simulink model "sim_final"  (R2023b)
settings: Solver=FixedStepAuto  StartTime=0.0  StopTime=10.0  RelTol=1e-3  EnableMultiTasking=on
libraries: raspberrypiAVlib x1
settings Model: Creator=Admin  LastModifiedBy=Admin
settings SolverCC: PositivePriorityOrder=on
settings OptimizationCC: EnhancedBackFolding=on  PassReuseOutputArgsAs=Individual arguments  ZeroExternalMemoryAtStartup=off  ZeroInternalMemoryAtStartup=off  MaxStackSize=64  OptimizeBlockOrder=speed  DifferentSizesBufferReuse=on  OptimizationCustomize=off  EfficientTunableParamExpr=on
settings DebuggingCC: ParameterTunabilityLossMsg=error
settings HardwareCC: ProdBitPerPointer=32  ProdBitPerSizeT=32  ProdBitPerPtrDiffT=32  ProdLargestAtomicInteger=Long  ProdLargestAtomicFloat=Double  ProdWordSize=32  ProdLongLongMode=on  ProdHWDeviceType=ARM Compatible->ARM Cortex  UseEmbeddedCoderFeatures=off  UseSimulinkCoderFeatures=off
settings RTWCC: Description=Embedded Coder  SystemTargetFile=ert.tlc  HardwareBoard=Raspberry Pi  TLCOptions="-aInlineSetEventsForThisBaseRateFcn=TLC_FALSE -aSuppressMultiTaskScheduler=TLC_FALSE  -aRateBasedStepFcn=0"  TemplateMakefile=ert_default_tmf  Toolchain=GNU GCC Embedded Linux  BuildConfiguration=Faster Runs
settings CodeAppCC: ForceParamTrailComments=on  IgnoreCustomStorageClasses=off  OperatorAnnotations=on  SimulinkDataObjDesc=on  SFDataObjDesc=on  InsertBlockDesc=on
settings ERTTargetCC: SupportNonInlinedSFcns=on  SupportVariableSizeSignals=on  ExtModeTransport=2  ExtModeStaticAlloc=on  ExtModeMexFile=ext_xcp  ExtModeIntrfLevel=Level2 - Open

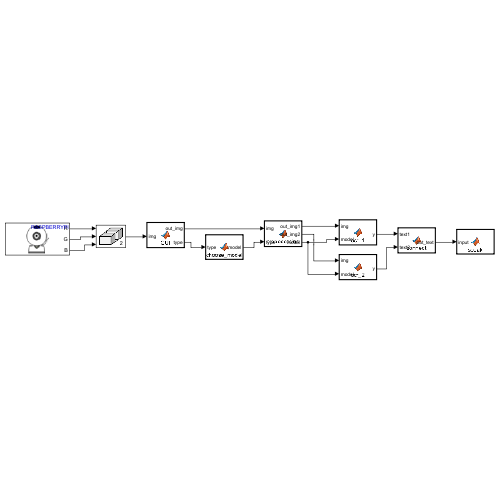
[thumbnail: Simulink's stored preview of the top-level diagram]
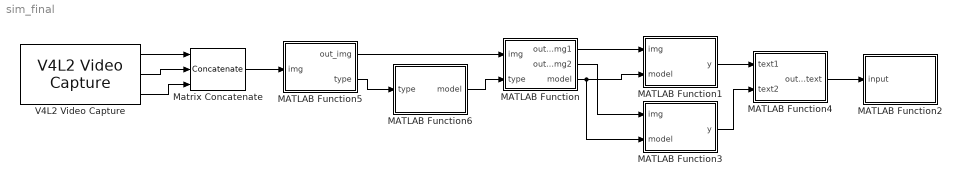
== system sim_final ==
  MATLAB Function : MATLAB Function  TreatAsAtomicUnit=on
  MATLAB Function1 : MATLAB Function  TreatAsAtomicUnit=on
  MATLAB Function2 : MATLAB Function  TreatAsAtomicUnit=on
  MATLAB Function3 : MATLAB Function  TreatAsAtomicUnit=on
  MATLAB Function4 : MATLAB Function  TreatAsAtomicUnit=on
  MATLAB Function5 : MATLAB Function  TreatAsAtomicUnit=on
  MATLAB Function6 : MATLAB Function  TreatAsAtomicUnit=on
  Matrix Concatenate : Concatenate  NumInputs=3  Mode=Multidimensional array  ConcatenateDimension=2
  V4L2 Video Capture : raspberrypiAVlib/V4L2 Video Capture  DeviceName=/dev/video0  Resolution=320x240  CustomResolution=[ 320, 240 ]  PixelFormat=RGB  SampleTime=0.1  pixelOrder=planar  simOutput=Colorbars  imSizeSelection=320x240  imSize=[640, 480]  roi=[0, 0, 640, 480]  m_devName='/dev/video0'  blockPlatform=LINUX  HorizontalFlip=off  VerticalFlip=off  Brightness=0.5  Saturation=0.5  Contrast=0.5  Sharpness=0.5  CameraPan=0  CameraTilt=0  CameraZoom=0.5  EnableManualFocus=on  ManualFocus=0.5
  wires:
  MATLAB Function/1(out_img1) -> MATLAB Function1/1(img)
  MATLAB Function5/2(type) -> MATLAB Function6/1(type)
  V4L2 Video Capture/1 -> Matrix Concatenate/1
  V4L2 Video Capture/2 -> Matrix Concatenate/2
  V4L2 Video Capture/3 -> Matrix Concatenate/3
  Matrix Concatenate/1 -> MATLAB Function5/1(img)
  MATLAB Function/2(out_img2) -> MATLAB Function3/1(img)
  MATLAB Function6/1(model) -> MATLAB Function/2(type)
  MATLAB Function5/1(out_img) -> MATLAB Function/1(img)
  MATLAB Function/3(model) -> MATLAB Function1/2(model), MATLAB Function3/2(model)
  MATLAB Function1/1(y) -> MATLAB Function4/1(text1)
  MATLAB Function3/1(y) -> MATLAB Function4/2(text2)
  MATLAB Function4/1(out_text) -> MATLAB Function2/1(input)

== matlab function sim_final/MATLAB Function1 ==
  data: img input; y output; model input
function y = ocr_1(img,model)

y = img;

== matlab function sim_final/MATLAB Function ==
  data: img input; out_img1 output; out_img2 output; type input; model output
function [out_img1,out_img2,model] = prepocessing(img,type)

out_img = img;

== matlab function sim_final/MATLAB Function2 ==
  data: input input
function speak(input)

y = u;

== matlab function sim_final/MATLAB Function3 ==
  data: img input; y output; model input
function y = ocr_2(img,model)

y = img;

== matlab function sim_final/MATLAB Function4 ==
  data: text1 input; out_text output; text2 input
function out_text = connect(text1,text2)

y = u;

== matlab function sim_final/MATLAB Function5 ==
  data: out_img output; img input; type output
function [out_img,type] = GUI(img)

y = u;

== matlab function sim_final/MATLAB Function6 ==
  data: type input; model output
function model = choose_model(type)

y = u;
